simulink model "DKHD_CH30_4_1_S"  (R2015a)
settings: Solver=ode45  StartTime=0.0  StopTime=2000  RelTol=1e-3
libraries: fuzblock x1, simulink x1
settings Model: CovSFcnEnable=off  Creator=URAGAN  LastModifiedBy=Admin
settings SolverCC: ZeroCrossControl=DisableAll
settings DataIOCC: MaxDataPoints=100000
settings DebuggingCC: SolverPrmCheckMsg=warning  MultiTaskDSMMsg=warning  MultiTaskCondExecSysMsg=none  FcnCallInpInsideContextMsg=EnableAllAsWarning  StrictBusMsg=ErrorOnBusTreatedAsVector

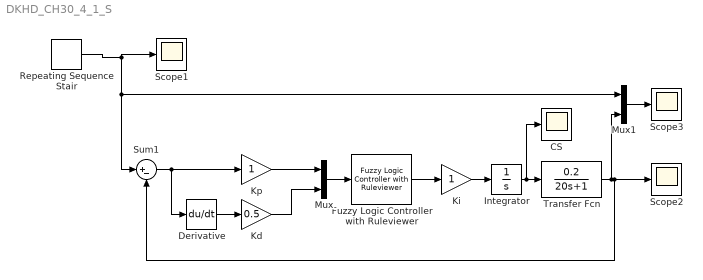
== system DKHD_CH30_4_1_S ==
  CS : Scope
  Derivative : Derivative
  Fuzzy Logic Controller with Ruleviewer : fuzblock/Fuzzy Logic  Controller  with Ruleviewer  fismatrix=DKHD_CH30_4_1_F  Ts=2
  Integrator : Integrator
  Kd : Gain  Gain=0.5
  Ki : Gain
  Kp : Gain
  Mux : Mux  Inputs=2
  Mux1 : Mux  Inputs=2
  Repeating Sequence Stair : simulink/Sources/Repeating Sequence Stair  OutValues=[100 150 75].'  tsamp=500  OutMin=[]  OutMax=[]  OutDataTypeStr=double  OutputDataTypeScalingMode=double  OutDataType=fixdt(0,8)  ConRadixGroup=Best Precision: Vector-wise  OutScaling=2^-12
  Scope1 : Scope
      settings: YMin=20  YMax=125
  Scope2 : Scope
      settings: TimeRange=10  YMin=-0.3  YMax=0.5  SaveName=ScopeData2
  Scope3 : Scope
      settings: YMin=0  YMax=170  SaveName=ScopeData3
  Sum1 : Sum  Inputs=|+-
  Transfer Fcn : TransferFcn  Numerator=[0.2]  Denominator=[20 1]
  wires:
  Transfer Fcn/1 -> Mux1/2, Sum1/2, Scope2/1
  Mux/1 -> Fuzzy Logic Controller with Ruleviewer/1
  Fuzzy Logic Controller with Ruleviewer/1 -> Ki/1
  Sum1/1 -> Derivative/1, Kp/1
  Ki/1 -> Integrator/1
  Kp/1 -> Mux/1
  Kd/1 -> Mux/2
  Repeating Sequence Stair/1 -> Sum1/1, Mux1/1, Scope1/1
  Integrator/1 -> CS/1, Transfer Fcn/1
  Derivative/1 -> Kd/1
  Mux1/1 -> Scope3/1
